simulink model "MotorControl_test"  (R2017a)
settings: Solver=FixedStepDiscrete  StartTime=0.0  StopTime=10.0  RelTol=1e-3
values from neighbouring files (symbols this model uses):
  Enum_MotorState : value not decoded    [MotorControl.sldd]
  PWMValue = 1000.0    [MotorControl.sldd]
undefined symbols (not defined in the file or in its folder): sigbuilder_block
libraries: simulink x5
settings Model: DataDictionary=MotorControl.sldd  Creator=Administrator  LastModifiedBy=Administrator
settings OptimizationCC: DefaultParameterBehavior=Inlined  PassReuseOutputArgsAs=Individual arguments
settings DebuggingCC: ParameterTunabilityLossMsg=error
settings SFSimCC: MATLABDynamicMemAlloc=off
settings RTWCC: SystemTargetFile=ert.tlc  GenCodeOnly=on  TemplateMakefile=ert_default_tmf  Description=Embedded Coder  GenerateReport=on  IncludeHyperlinkInReport=on  LaunchReport=on  GenerateTraceInfo=on  GenerateTraceReport=on  GenerateTraceReportSl=on  GenerateTraceReportSf=on  GenerateTraceReportEml=on
settings CodeAppCC: ForceParamTrailComments=on  IgnoreCustomStorageClasses=off  OperatorAnnotations=on  SimulinkDataObjDesc=on  SFDataObjDesc=on  MATLABFcnDesc=on  InsertBlockDesc=on  MATLABSourceComments=on
settings ERTTargetCC: TargetLangStandard=C99 (ISO)  InlinedParameterPlacement=NonHierarchical  ERTCustomFileTemplate=example_file_process.tlc

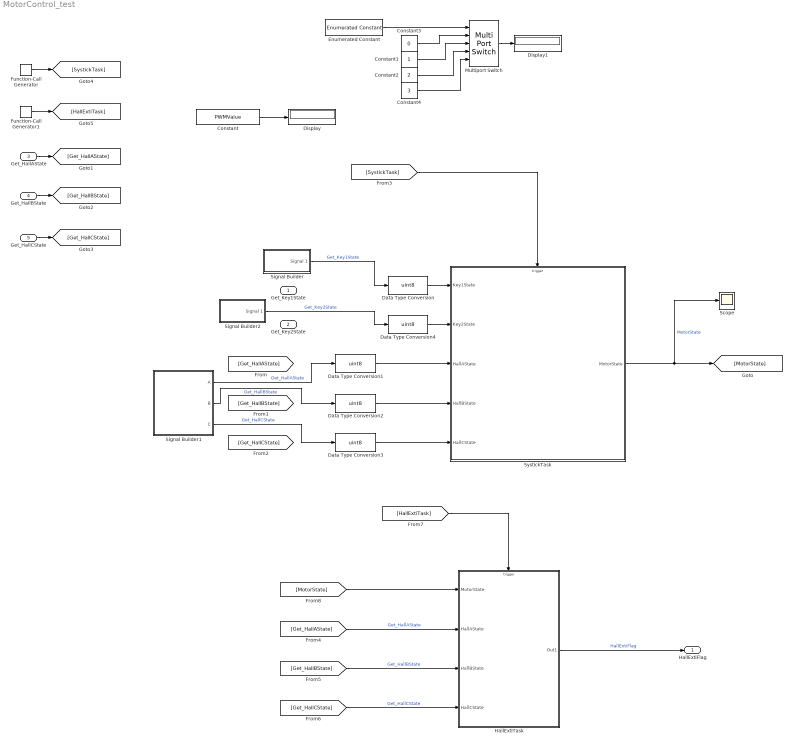
== system MotorControl_test ==
  Get_Key1State : Inport
  Get_Key2State : Inport  Port=2
  Get_HallAState : Inport  Port=3
  Get_HallBState : Inport  Port=4
  Get_HallCState : Inport  Port=5
  Constant : Constant  Value=PWMValue
  Constant1 : Constant  OutDataTypeStr=uint8
  Constant2 : Constant  Value=2  OutDataTypeStr=uint8
  Constant3 : Constant  Value=0  OutDataTypeStr=uint8
  Constant4 : Constant  Value=3  OutDataTypeStr=uint8
  Data Type Conversion{,1..4} (5 alike) : DataTypeConversion  OutDataTypeStr=uint8
  Display : Display
  Display1 : Display
  Enumerated Constant : simulink/Sources/Enumerated Constant  OutDataTypeStr=Enum: Enum_MotorState  Value=Enum_MotorState.Run  SampleTime=inf
      settings: SourceProductName=Simulink
  Function-Call Generator : simulink/Ports & Subsystems/Function-Call Generator  sample_time=0.001  numberOfIterations=1
  Function-Call Generator1 : simulink/Ports & Subsystems/Function-Call Generator  sample_time=1  numberOfIterations=1
  HallExtiTask : Subsystem  TreatAsAtomicUnit=on  RTWFcnName=HallExtiTask
      settings: RTWSystemCode=Nonreusable function  RTWFcnNameOpts=User specified  RTWFileNameOpts=Use function name
  Multiport Switch : MultiPortSwitch  DataPortOrder=Specify indices  DataPortIndices={Enum_MotorState.Init,Enum_MotorState.Stop,Enum_MotorState.Start,Enum_MotorState.Run}
  Scope : Scope
  Signal Builder : Subsystem  Tag=STV Subsys  LoadFcn=sigbuilder_block('load');  StartFcn=sigbuilder_block('start');  StopFcn=sigbuilder_block('stop');  ClipboardFcn=sigbuilder_block('clipboard');  mask(Sigbuilder block){tuvar=[0:10]}
      mask help: Simulink:masks:SigbuilderBlock_MD
      mask init:
      | if ~strcmp(get_param(bdroot(gcbh),'SimulationStatus'),'stopped') tuvar = sigbuilder_block('maskInit'); end
      settings: CopyFcn=sigbuilder_block('copy');  DeleteFcn=sigbuilder_block('delete');  ModelCloseFcn=sigbuilder_block('modelClose');  PreSaveFcn=sigbuilder_block('preSave');  PauseFcn=sigbuilder_block('pause');  ContinueFcn=sigbuilder_block('continue');  NameChangeFcn=sigbuilder_block('namechange');  OpenFcn=sigbuilder_block('open',[437.6 199.2 550.4 400 ]);  CloseFcn=sigbuilder_block('close');
      mask Display: plot(0, 0, 100, 100,[2, 2, 32, 32, 2], [68, 8, 8, 68, 68],[32, 2], [38, 38], [32, 19, 2],[53, 60, 44], [32, 17, 17, 2],[16, 16, 31, 31]);txt = getActiveGroup(gcbh);text(2, 100, txt,'verticalAlignment', 'top');
  Signal Builder1 : Subsystem  Tag=STV Subsys  LoadFcn=sigbuilder_block('load');  StartFcn=sigbuilder_block('start');  StopFcn=sigbuilder_block('stop');  ClipboardFcn=sigbuilder_block('clipboard');  mask(Sigbuilder block){tuvar=[0:10]}
      mask help: Simulink:masks:SigbuilderBlock_MD
      mask init:
      | if ~strcmp(get_param(bdroot(gcbh),'SimulationStatus'),'stopped') tuvar = sigbuilder_block('maskInit'); end
      settings: CopyFcn=sigbuilder_block('copy');  DeleteFcn=sigbuilder_block('delete');  ModelCloseFcn=sigbuilder_block('modelClose');  PreSaveFcn=sigbuilder_block('preSave');  PauseFcn=sigbuilder_block('pause');  ContinueFcn=sigbuilder_block('continue');  NameChangeFcn=sigbuilder_block('namechange');  OpenFcn=sigbuilder_block('open',[437.6 199.2 550.4 400 ]);  CloseFcn=sigbuilder_block('close');
      mask Display: plot(0, 0, 100, 100,[2, 2, 32, 32, 2], [68, 8, 8, 68, 68],[32, 2], [38, 38], [32, 19, 2],[53, 60, 44], [32, 17, 17, 2],[16, 16, 31, 31]);txt = getActiveGroup(gcbh);text(2, 100, txt,'verticalAlignment', 'top');
  Signal Builder2 : Subsystem  Tag=STV Subsys  LoadFcn=sigbuilder_block('load');  StartFcn=sigbuilder_block('start');  StopFcn=sigbuilder_block('stop');  ClipboardFcn=sigbuilder_block('clipboard');  mask(Sigbuilder block){tuvar=[0:10]}
      mask help: Simulink:masks:SigbuilderBlock_MD
      mask init:
      | if ~strcmp(get_param(bdroot(gcbh),'SimulationStatus'),'stopped') tuvar = sigbuilder_block('maskInit'); end
      settings: CopyFcn=sigbuilder_block('copy');  DeleteFcn=sigbuilder_block('delete');  ModelCloseFcn=sigbuilder_block('modelClose');  PreSaveFcn=sigbuilder_block('preSave');  PauseFcn=sigbuilder_block('pause');  ContinueFcn=sigbuilder_block('continue');  NameChangeFcn=sigbuilder_block('namechange');  OpenFcn=sigbuilder_block('open',[437.6 199.2 550.4 400 ]);  CloseFcn=sigbuilder_block('close');
      mask Display: plot(0, 0, 100, 100,[2, 2, 32, 32, 2], [68, 8, 8, 68, 68],[32, 2], [38, 38], [32, 19, 2],[53, 60, 44], [32, 17, 17, 2],[16, 16, 31, 31]);txt = getActiveGroup(gcbh);text(2, 100, txt,'verticalAlignment', 'top');
  SystickTask : Subsystem  TreatAsAtomicUnit=on  RTWFcnName=SystickTask
      settings: RTWSystemCode=Nonreusable function  RTWFcnNameOpts=User specified  RTWFileNameOpts=Use function name
  HallExtiFlag : Outport
  wires:
  SystickTask/1(MotorState) -> Scope/1, [MotorState]  "MotorState"
  HallExtiTask/1(Out1) -> HallExtiFlag/1  "HallExtiFlag"
  [SystickTask] -> SystickTask/Trigger
  Signal Builder1/1(A) -> Data Type Conversion1/1  "Get_HallAState"
  Signal Builder1/3(C) -> Data Type Conversion3/1  "Get_HallCState"
  Signal Builder1/2(B) -> Data Type Conversion2/1  "Get_HallBState"
  Signal Builder2/1(Signal 1) -> Data Type Conversion4/1  "Get_Key2State"
  Signal Builder/1(Signal 1) -> Data Type Conversion/1  "Get_Key1State"
  [HallExtiTask] -> HallExtiTask/Trigger
  [Get_HallCState] -> HallExtiTask/4(HallCState)  "Get_HallCState"
  [Get_HallBState] -> HallExtiTask/3(HallBState)  "Get_HallBState"
  [Get_HallAState] -> HallExtiTask/2(HallAState)  "Get_HallAState"
  [MotorState] -> HallExtiTask/1(MotorState)
  Get_HallAState/1 -> [Get_HallAState]
  Get_HallBState/1 -> [Get_HallBState]
  Get_HallCState/1 -> [Get_HallCState]
  Function-Call Generator/1 -> [SystickTask]
  Function-Call Generator1/1 -> [HallExtiTask]
  Data Type Conversion/1 -> SystickTask/1(Key1State)
  Data Type Conversion1/1 -> SystickTask/3(HallAState)
  Data Type Conversion2/1 -> SystickTask/4(HallBState)
  Data Type Conversion3/1 -> SystickTask/5(HallCState)
  Data Type Conversion4/1 -> SystickTask/2(Key2State)
  Constant/1 -> Display/1
  Constant3/1 -> Multiport Switch/2
  Enumerated Constant/1 -> Multiport Switch/1
  Constant1/1 -> Multiport Switch/3
  Constant2/1 -> Multiport Switch/4
  Constant4/1 -> Multiport Switch/5
  Multiport Switch/1 -> Display1/1

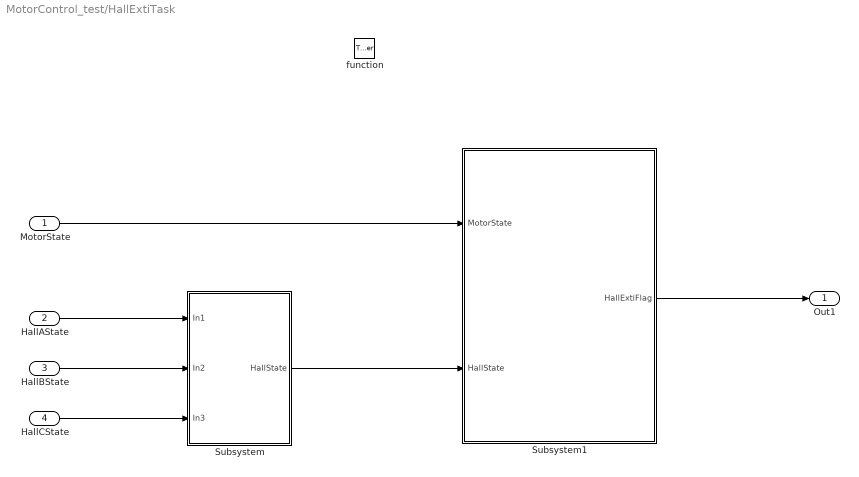
== system MotorControl_test/HallExtiTask ==
  MotorState : Inport
  HallAState : Inport  Port=2
  HallBState : Inport  Port=3
  HallCState : Inport  Port=4
  function : TriggerPort  TriggerType=function-call  VariantControl=Variant
  Subsystem : Subsystem
  Subsystem1 : Subsystem
  Out1 : Outport
  wires:
  HallBState/1 -> Subsystem/2(In2)
  HallAState/1 -> Subsystem/1(In1)
  HallCState/1 -> Subsystem/3(In3)
  MotorState/1 -> Subsystem1/1(MotorState)
  Subsystem/1(HallState) -> Subsystem1/2(HallState)
  Subsystem1/1(HallExtiFlag) -> Out1/1

== system MotorControl_test/Signal Builder ==
  Demux : Demux  Tag=STV Demux  Outputs=1
  FromWs : FromWorkspace  Tag=STV FromWs  VariableName=tuvar  SampleTime=0
      SigBuilderData=|
      | common.afterFinalStr = 'Extrapolate'
      | common.sampleTime = 0
      | dataSet.timeRange = [0 10]
      | dataSet.name = 'Group 1'
      | sbobj.Groups.Name = 'Group 1'
      | sbobj.Groups.Signals.Name = 'Signal 1'
      | sbobj.Groups.Signals.XData = [0 4 4 6 6 10]
      | sbobj.Groups.Signals.YData = [0 0 1 1 0 0]
  Signal 1 : Outport  Tag=STV Outport
  wires:
  Demux/1 -> Signal 1/1
  FromWs/1 -> Demux/1

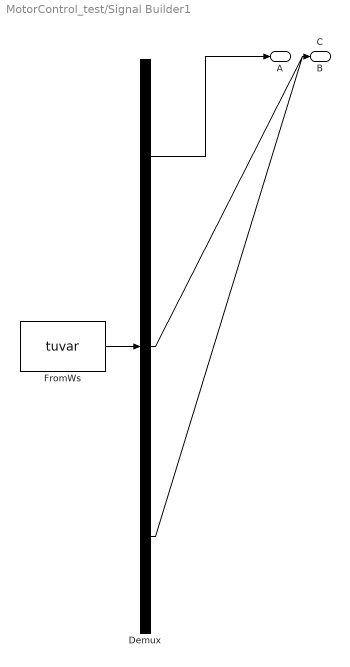
== system MotorControl_test/Signal Builder1 ==
  Demux : Demux  Tag=STV Demux  Outputs=3
  FromWs : FromWorkspace  Tag=STV FromWs  VariableName=tuvar  SampleTime=0
      SigBuilderData=|
      | common.afterFinalStr = 'Extrapolate'
      | common.sampleTime = 0
      | dataSet.timeRange = [0 7.999]
      | dataSet.name = 'Sheet1'
      | sbobj.Groups.Name = 'Sheet1'
      | sbobj.Groups.Signals(1).Name = 'A'
      | sbobj.Groups.Signals(1).XData = [0 4.999 5 5.499 5.5 5.999 6 6.499 6.5 6.999 7 7.499 7.5 7.999]
      | sbobj.Groups.Signals(1).YData = [0 0 1 1 1 1 1 1 0 0 0 0 0 0]
      | sbobj.Groups.Signals(2).Name = 'B'
      | sbobj.Groups.Signals(2).XData = [0 4.999 5 5.499 5.5 5.999 6 6.499 6.5 6.999 7 7.499 7.5 7.999]
      | sbobj.Groups.Signals(2).YData = [0 0 0 0 0 0 1 1 1 1 1 1 0 0]
      | sbobj.Groups.Signals(3).Name = 'C'
      | sbobj.Groups.Signals(3).XData = [0 4.999 5 5.499 5.5 5.999 6 6.499 6.5 6.999 7 7.499 7.5 7.999]
      | sbobj.Groups.Signals(3).YData = [0 0 1 1 0 0 0 0 0 0 1 1 1 1]
      | sbobj.Groups.TimeRange = [0 7.999]
  A : Outport  Tag=STV Outport
  B : Outport  Tag=STV Outport  Port=2
  C : Outport  Tag=STV Outport  Port=3
  wires:
  FromWs/1 -> Demux/1
  Demux/1 -> A/1
  Demux/2 -> B/1
  Demux/3 -> C/1

== system MotorControl_test/Signal Builder2 ==
  Demux : Demux  Tag=STV Demux  Outputs=1
  FromWs : FromWorkspace  Tag=STV FromWs  VariableName=tuvar  SampleTime=0
      SigBuilderData=|
      | common.afterFinalStr = 'Extrapolate'
      | common.sampleTime = 0
      | dataSet.timeRange = [0 10]
      | dataSet.name = 'Group 1'
      | sbobj.Groups.Name = 'Group 1'
      | sbobj.Groups.Signals.Name = 'Signal 1'
      | sbobj.Groups.Signals.XData = [0 9 9 9.76 9.76 10]
      | sbobj.Groups.Signals.YData = [0 0 1 1 0 0]
  Signal 1 : Outport  Tag=STV Outport
  wires:
  FromWs/1 -> Demux/1
  Demux/1 -> Signal 1/1

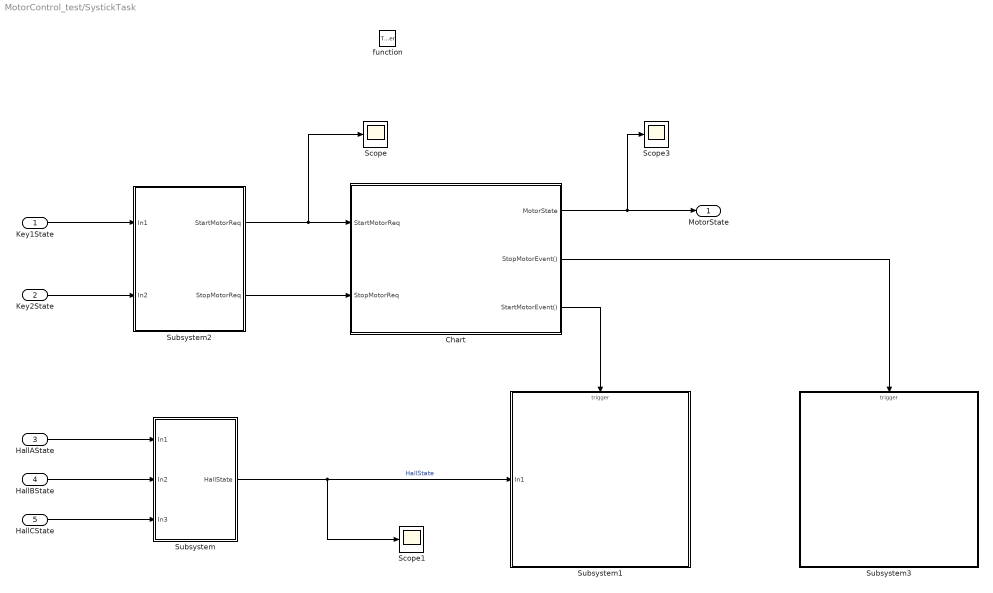
== system MotorControl_test/SystickTask ==
  Key1State : Inport
  Key2State : Inport  Port=2
  HallAState : Inport  Port=3
  HallBState : Inport  Port=4
  HallCState : Inport  Port=5
  function : TriggerPort  TriggerType=function-call  VariantControl=Variant
  Chart : Stateflow chart  TreatAsAtomicUnit=on
  Scope : Scope
  Scope1 : Scope
  Scope3 : Scope
  Subsystem : Subsystem
  Subsystem1 : Subsystem
  Subsystem2 : Subsystem
  Subsystem3 : Subsystem
      settings: RTWSystemCode=Nonreusable function
  MotorState : Outport
  wires:
  Key1State/1 -> Subsystem2/1(In1)
  Key2State/1 -> Subsystem2/2(In2)
  Subsystem2/1(StartMotorReq) -> Scope/1, Chart/1(StartMotorReq)
  Subsystem2/2(StopMotorReq) -> Chart/2(StopMotorReq)
  Chart/1(MotorState) -> Scope3/1, MotorState/1
  HallAState/1 -> Subsystem/1(In1)
  HallBState/1 -> Subsystem/2(In2)
  HallCState/1 -> Subsystem/3(In3)
  Subsystem/1(HallState) -> Subsystem1/1(In1), Scope1/1  "HallState"
  Chart/2(StopMotorEvent()) -> Subsystem3/Trigger
  Chart/3(StartMotorEvent()) -> Subsystem1/Trigger

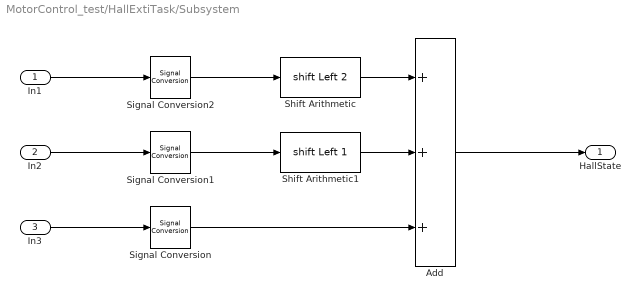
== system MotorControl_test/HallExtiTask/Subsystem ==
  In1 : Inport
  In2 : Inport  Port=2
  In3 : Inport  Port=3
  Add : Sum  Inputs=+++
  Shift Arithmetic : ArithShift  BitShiftNumber=2  BitShiftDirection=Left
  Shift Arithmetic1 : ArithShift  BitShiftNumber=1  BitShiftDirection=Left
  Signal Conversion : SignalConversion  OverrideOpt=off
  Signal Conversion1 : SignalConversion  OverrideOpt=off
  Signal Conversion2 : SignalConversion  OverrideOpt=on
  HallState : Outport
  wires:
  Add/1 -> HallState/1
  Signal Conversion/1 -> Add/3
  In3/1 -> Signal Conversion/1
  Signal Conversion1/1 -> Shift Arithmetic1/1
  Signal Conversion2/1 -> Shift Arithmetic/1
  Shift Arithmetic/1 -> Add/1
  In1/1 -> Signal Conversion2/1
  In2/1 -> Signal Conversion1/1
  Shift Arithmetic1/1 -> Add/2

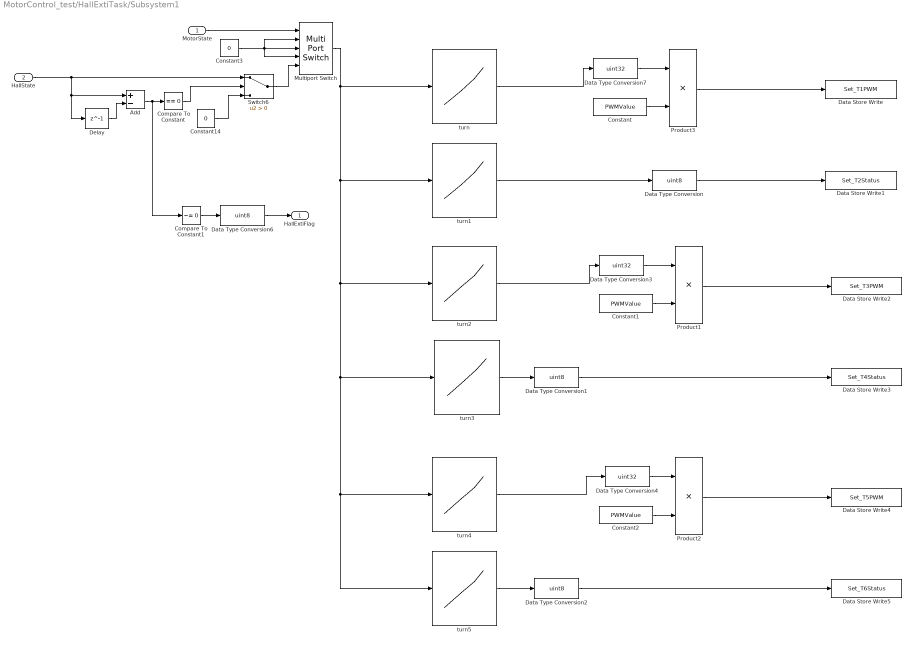
== system MotorControl_test/HallExtiTask/Subsystem1 ==
  MotorState : Inport
  HallState : Inport  Port=2
  Add : Sum  Inputs=+-
  Compare To Constant : simulink/Logic and Bit Operations/Compare To Constant  relop===  const=0  OutDataTypeStr=boolean
  Compare To Constant1 : simulink/Logic and Bit Operations/Compare To Constant  relop=~=  const=0  OutDataTypeStr=boolean
  Constant : Constant  Value=PWMValue
  Constant1 : Constant  Value=PWMValue
  Constant14 : Constant  Value=0  OutDataTypeStr=uint8
  Constant2 : Constant  Value=PWMValue
  Constant3 : Constant  Value=0  OutDataTypeStr=uint8
  Data Store Write : DataStoreWrite  DataStoreName=Set_T1PWM
  Data Store Write1 : DataStoreWrite  DataStoreName=Set_T2Status
  Data Store Write2 : DataStoreWrite  DataStoreName=Set_T3PWM
  Data Store Write3 : DataStoreWrite  DataStoreName=Set_T4Status
  Data Store Write4 : DataStoreWrite  DataStoreName=Set_T5PWM
  Data Store Write5 : DataStoreWrite  DataStoreName=Set_T6Status
  Data Type Conversion{,1..2,6} (4 alike) : DataTypeConversion  OutDataTypeStr=uint8
  Data Type Conversion3 : DataTypeConversion  OutDataTypeStr=uint32
  Data Type Conversion4 : DataTypeConversion  OutDataTypeStr=uint32
  Data Type Conversion7 : DataTypeConversion  OutDataTypeStr=uint32
  Delay : Delay  DelayLength=1  InitialCondition=0
  Multiport Switch : MultiPortSwitch  DataPortOrder=Specify indices  DataPortIndices={Enum_MotorState.Init,Enum_MotorState.Stop,Enum_MotorState.Start,Enum_MotorState.Run}
  Product1 : Product  OutDataTypeStr=uint32
  Product2 : Product  OutDataTypeStr=uint32
  Product3 : Product  OutDataTypeStr=uint32
  Switch6 : Switch  Criteria=u2 > Threshold
  turn : Lookup_n-D  NumberOfTableDimensions=1  BreakpointsForDimension1=[0 1 2 3 4 5 6]  Table=[0 0 0 0 1 1 0]  InterpMethod=Nearest  InternalRulePriority=Speed  RndMeth=Simplest  InputSameDT=on
  turn1 : Lookup_n-D  NumberOfTableDimensions=1  BreakpointsForDimension1=[0 1 2 3 4 5 6]  Table=[0 0 1 1 0 0 0 ]  InterpMethod=Nearest  InternalRulePriority=Speed  RndMeth=Simplest  InputSameDT=on
  turn2 : Lookup_n-D  NumberOfTableDimensions=1  BreakpointsForDimension1=[0 1 2 3 4 5 6]  Table=[0 0 1 0 0 0 1]  InterpMethod=Nearest  InternalRulePriority=Speed  RndMeth=Simplest  InputSameDT=on
  turn3 : Lookup_n-D  NumberOfTableDimensions=1  BreakpointsForDimension1=[0 1 2 3 4 5 6]  Table=[0 1 0 0 0 1 0]  InterpMethod=Nearest  InternalRulePriority=Speed  RndMeth=Simplest  InputSameDT=on
  turn4 : Lookup_n-D  NumberOfTableDimensions=1  BreakpointsForDimension1=[0 1 2 3 4 5 6]  Table=[0 1 0 1 0 0 0]  InterpMethod=Nearest  InternalRulePriority=Speed  RndMeth=Simplest  InputSameDT=on
  turn5 : Lookup_n-D  NumberOfTableDimensions=1  BreakpointsForDimension1=[0 1 2 3 4 5 6]  Table=[0 0 0 0 1 0 1]  InterpMethod=Nearest  InternalRulePriority=Speed  RndMeth=Simplest  InputSameDT=on
  HallExtiFlag : Outport
  wires:
  Constant2/1 -> Product2/2
  turn5/1 -> Data Type Conversion2/1
  Product2/1 -> Data Store Write4/1
  Data Type Conversion2/1 -> Data Store Write5/1
  turn4/1 -> Data Type Conversion4/1
  turn1/1 -> Data Type Conversion/1
  Multiport Switch/1 -> turn/1, turn4/1, turn5/1, turn3/1, turn2/1, turn1/1
  Data Type Conversion/1 -> Data Store Write1/1
  turn3/1 -> Data Type Conversion1/1
  Constant1/1 -> Product1/2
  turn2/1 -> Data Type Conversion3/1
  Product1/1 -> Data Store Write2/1
  Data Type Conversion1/1 -> Data Store Write3/1
  Product3/1 -> Data Store Write/1
  turn/1 -> Data Type Conversion7/1
  Constant/1 -> Product3/2
  Compare To Constant/1 -> Switch6/2
  Delay/1 -> Add/2
  HallState/1 -> Add/1, Delay/1, Switch6/1
  Constant14/1 -> Switch6/3
  Add/1 -> Compare To Constant1/1, Compare To Constant/1
  MotorState/1 -> Multiport Switch/1
  Switch6/1 -> Multiport Switch/5
  Constant3/1 -> Multiport Switch/2, Multiport Switch/3, Multiport Switch/4
  Compare To Constant1/1 -> Data Type Conversion6/1
  Data Type Conversion6/1 -> HallExtiFlag/1
  Data Type Conversion7/1 -> Product3/1
  Data Type Conversion3/1 -> Product1/1
  Data Type Conversion4/1 -> Product2/1

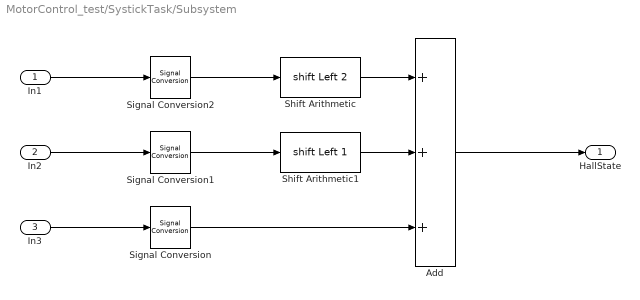
== system MotorControl_test/SystickTask/Subsystem ==
  In1 : Inport
  In2 : Inport  Port=2
  In3 : Inport  Port=3
  Add : Sum  Inputs=+++
  Shift Arithmetic : ArithShift  BitShiftNumber=2  BitShiftDirection=Left
  Shift Arithmetic1 : ArithShift  BitShiftNumber=1  BitShiftDirection=Left
  Signal Conversion : SignalConversion  OverrideOpt=off
  Signal Conversion1 : SignalConversion  OverrideOpt=off
  Signal Conversion2 : SignalConversion  OverrideOpt=off
  HallState : Outport
  wires:
  Add/1 -> HallState/1
  Signal Conversion/1 -> Add/3
  In3/1 -> Signal Conversion/1
  Signal Conversion1/1 -> Shift Arithmetic1/1
  Signal Conversion2/1 -> Shift Arithmetic/1
  Shift Arithmetic/1 -> Add/1
  In1/1 -> Signal Conversion2/1
  In2/1 -> Signal Conversion1/1
  Shift Arithmetic1/1 -> Add/2

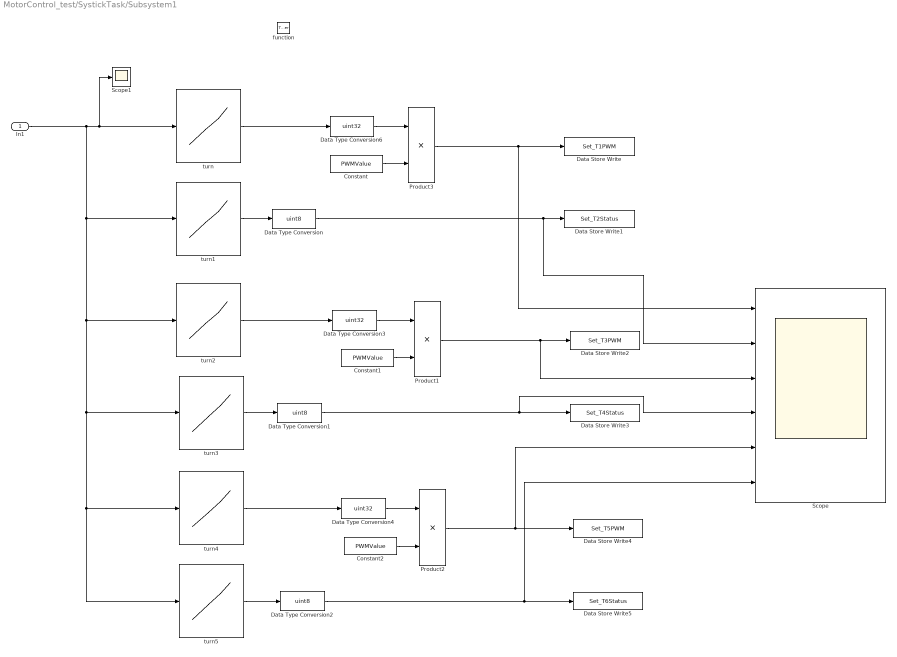
== system MotorControl_test/SystickTask/Subsystem1 ==
  In1 : Inport
  function : TriggerPort  TriggerType=function-call  VariantControl=Variant
  Constant : Constant  Value=PWMValue
  Constant1 : Constant  Value=PWMValue
  Constant2 : Constant  Value=PWMValue
  Data Store Write : DataStoreWrite  DataStoreName=Set_T1PWM
  Data Store Write1 : DataStoreWrite  DataStoreName=Set_T2Status
  Data Store Write2 : DataStoreWrite  DataStoreName=Set_T3PWM
  Data Store Write3 : DataStoreWrite  DataStoreName=Set_T4Status
  Data Store Write4 : DataStoreWrite  DataStoreName=Set_T5PWM
  Data Store Write5 : DataStoreWrite  DataStoreName=Set_T6Status
  Data Type Conversion : DataTypeConversion  OutDataTypeStr=uint8
  Data Type Conversion1 : DataTypeConversion  OutDataTypeStr=uint8
  Data Type Conversion2 : DataTypeConversion  OutDataTypeStr=uint8
  Data Type Conversion3 : DataTypeConversion  OutDataTypeStr=uint32
  Data Type Conversion4 : DataTypeConversion  OutDataTypeStr=uint32
  Data Type Conversion6 : DataTypeConversion  OutDataTypeStr=uint32
  Product1 : Product  OutDataTypeStr=uint32
  Product2 : Product  OutDataTypeStr=uint32
  Product3 : Product  OutDataTypeStr=uint32
  Scope : Scope  NumInputPorts=6
  Scope1 : Scope
  turn : Lookup_n-D  NumberOfTableDimensions=1  BreakpointsForDimension1=[1 2 3 4 5 6]  Table=[0 0 0 1 1 0]  InterpMethod=Nearest  InternalRulePriority=Speed  RndMeth=Simplest  InputSameDT=on
  turn1 : Lookup_n-D  NumberOfTableDimensions=1  BreakpointsForDimension1=[1 2 3 4 5 6]  Table=[0 1 1 0 0 0 ]  InterpMethod=Nearest  InternalRulePriority=Speed  RndMeth=Simplest  InputSameDT=on
  turn2 : Lookup_n-D  NumberOfTableDimensions=1  BreakpointsForDimension1=[1 2 3 4 5 6]  Table=[0 1 0 0 0 1]  InterpMethod=Nearest  InternalRulePriority=Speed  RndMeth=Simplest  InputSameDT=on
  turn3 : Lookup_n-D  NumberOfTableDimensions=1  BreakpointsForDimension1=[1 2 3 4 5 6]  Table=[1 0 0 0 1 0]  InterpMethod=Nearest  InternalRulePriority=Speed  RndMeth=Simplest  InputSameDT=on
  turn4 : Lookup_n-D  NumberOfTableDimensions=1  BreakpointsForDimension1=[1 2 3 4 5 6]  Table=[1 0 1 0 0 0]  InterpMethod=Nearest  InternalRulePriority=Speed  RndMeth=Simplest  InputSameDT=on
  turn5 : Lookup_n-D  NumberOfTableDimensions=1  BreakpointsForDimension1=[1 2 3 4 5 6]  Table=[0 0 0 1 0 1]  InterpMethod=Nearest  InternalRulePriority=Speed  RndMeth=Simplest  InputSameDT=on
  wires:
  Constant2/1 -> Product2/2
  turn5/1 -> Data Type Conversion2/1
  Product2/1 -> Scope/5, Data Store Write4/1
  Data Type Conversion2/1 -> Scope/6, Data Store Write5/1
  turn4/1 -> Data Type Conversion4/1
  turn1/1 -> Data Type Conversion/1
  In1/1 -> turn1/1, turn3/1, turn4/1, turn5/1, turn2/1, Scope1/1, turn/1
  Data Type Conversion/1 -> Scope/2, Data Store Write1/1
  turn3/1 -> Data Type Conversion1/1
  Constant1/1 -> Product1/2
  turn2/1 -> Data Type Conversion3/1
  Product1/1 -> Scope/3, Data Store Write2/1
  Data Type Conversion1/1 -> Scope/4, Data Store Write3/1
  Product3/1 -> Scope/1, Data Store Write/1
  turn/1 -> Data Type Conversion6/1
  Constant/1 -> Product3/2
  Data Type Conversion6/1 -> Product3/1
  Data Type Conversion3/1 -> Product1/1
  Data Type Conversion4/1 -> Product2/1

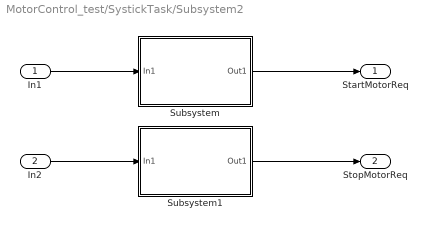
== system MotorControl_test/SystickTask/Subsystem2 ==
  In1 : Inport
  In2 : Inport  Port=2
  Subsystem : Subsystem
  Subsystem1 : Subsystem
  StartMotorReq : Outport
  StopMotorReq : Outport  Port=2
  wires:
  Subsystem/1(Out1) -> StartMotorReq/1
  Subsystem1/1(Out1) -> StopMotorReq/1
  In2/1 -> Subsystem1/1(In1)
  In1/1 -> Subsystem/1(In1)

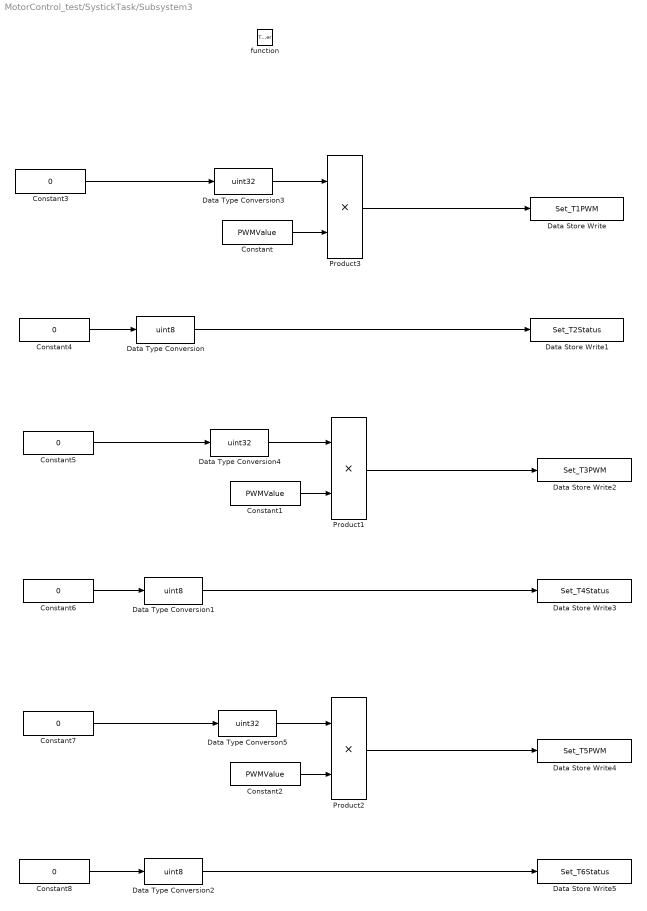
== system MotorControl_test/SystickTask/Subsystem3 ==
  function : TriggerPort  TriggerType=function-call  VariantControl=Variant
  Constant : Constant  Value=PWMValue
  Constant1 : Constant  Value=PWMValue
  Constant2 : Constant  Value=PWMValue
  Constant{3..8} (6 alike) : Constant  Value=0
  Data Store Write : DataStoreWrite  DataStoreName=Set_T1PWM
  Data Store Write1 : DataStoreWrite  DataStoreName=Set_T2Status
  Data Store Write2 : DataStoreWrite  DataStoreName=Set_T3PWM
  Data Store Write3 : DataStoreWrite  DataStoreName=Set_T4Status
  Data Store Write4 : DataStoreWrite  DataStoreName=Set_T5PWM
  Data Store Write5 : DataStoreWrite  DataStoreName=Set_T6Status
  Data Type Conversion : DataTypeConversion  OutDataTypeStr=uint8
  Data Type Conversion1 : DataTypeConversion  OutDataTypeStr=uint8
  Data Type Conversion2 : DataTypeConversion  OutDataTypeStr=uint8
  Data Type Conversion3 : DataTypeConversion  OutDataTypeStr=uint32
  Data Type Conversion4 : DataTypeConversion  OutDataTypeStr=uint32
  Data Type Converson5 : DataTypeConversion  OutDataTypeStr=uint32
  Product1 : Product  OutDataTypeStr=uint32
  Product2 : Product  OutDataTypeStr=uint32
  Product3 : Product  OutDataTypeStr=uint32
  wires:
  Constant/1 -> Product3/2
  Constant3/1 -> Data Type Conversion3/1
  Product3/1 -> Data Store Write/1
  Data Type Conversion1/1 -> Data Store Write3/1
  Product1/1 -> Data Store Write2/1
  Constant5/1 -> Data Type Conversion4/1
  Constant1/1 -> Product1/2
  Constant6/1 -> Data Type Conversion1/1
  Data Type Conversion/1 -> Data Store Write1/1
  Constant4/1 -> Data Type Conversion/1
  Constant7/1 -> Data Type Converson5/1
  Data Type Conversion2/1 -> Data Store Write5/1
  Product2/1 -> Data Store Write4/1
  Constant8/1 -> Data Type Conversion2/1
  Constant2/1 -> Product2/2
  Data Type Conversion3/1 -> Product3/1
  Data Type Conversion4/1 -> Product1/1
  Data Type Converson5/1 -> Product2/1

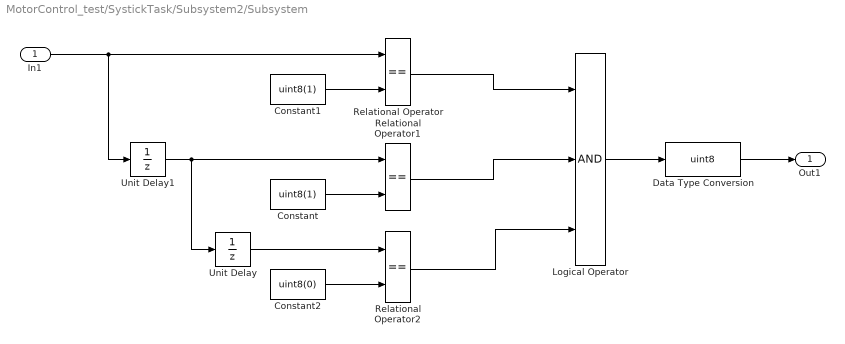
== system MotorControl_test/SystickTask/Subsystem2/Subsystem ==
  In1 : Inport
  Constant : Constant  Value=uint8(1)
  Constant1 : Constant  Value=uint8(1)
  Constant2 : Constant  Value=uint8(0)
  Data Type Conversion : DataTypeConversion  OutDataTypeStr=uint8
  Logical Operator : Logic  Inputs=3  AllPortsSameDT=off  OutDataTypeStr=boolean
  Relational Operator : RelationalOperator  Operator===  OutDataTypeStr=boolean  RndMeth=Simplest
  Relational Operator1 : RelationalOperator  Operator===  OutDataTypeStr=boolean  RndMeth=Simplest
  Relational Operator2 : RelationalOperator  Operator===  OutDataTypeStr=boolean  RndMeth=Simplest
  Unit Delay : UnitDelay  SampleTime=-1
  Unit Delay1 : UnitDelay  SampleTime=-1
  Out1 : Outport
  wires:
  Constant2/1 -> Relational Operator2/2
  Unit Delay1/1 -> Unit Delay/1, Relational Operator1/1
  Constant1/1 -> Relational Operator/2
  Relational Operator2/1 -> Logical Operator/3
  Relational Operator1/1 -> Logical Operator/2
  Relational Operator/1 -> Logical Operator/1
  Constant/1 -> Relational Operator1/2
  In1/1 -> Unit Delay1/1, Relational Operator/1
  Unit Delay/1 -> Relational Operator2/1
  Logical Operator/1 -> Data Type Conversion/1
  Data Type Conversion/1 -> Out1/1

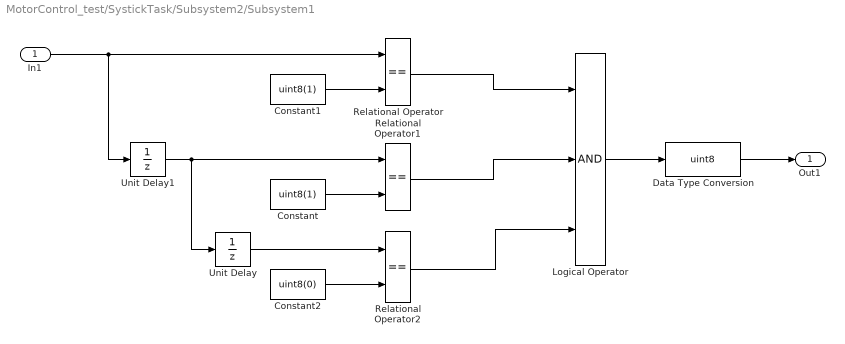
== system MotorControl_test/SystickTask/Subsystem2/Subsystem1 ==
  In1 : Inport
  Constant : Constant  Value=uint8(1)
  Constant1 : Constant  Value=uint8(1)
  Constant2 : Constant  Value=uint8(0)
  Data Type Conversion : DataTypeConversion  OutDataTypeStr=uint8
  Logical Operator : Logic  Inputs=3  AllPortsSameDT=off  OutDataTypeStr=boolean
  Relational Operator : RelationalOperator  Operator===  OutDataTypeStr=boolean  RndMeth=Simplest
  Relational Operator1 : RelationalOperator  Operator===  OutDataTypeStr=boolean  RndMeth=Simplest
  Relational Operator2 : RelationalOperator  Operator===  OutDataTypeStr=boolean  RndMeth=Simplest
  Unit Delay : UnitDelay  SampleTime=-1
  Unit Delay1 : UnitDelay  SampleTime=-1
  Out1 : Outport
  wires:
  Data Type Conversion/1 -> Out1/1
  Logical Operator/1 -> Data Type Conversion/1
  Unit Delay/1 -> Relational Operator2/1
  In1/1 -> Relational Operator/1, Unit Delay1/1
  Constant/1 -> Relational Operator1/2
  Relational Operator/1 -> Logical Operator/1
  Relational Operator1/1 -> Logical Operator/2
  Relational Operator2/1 -> Logical Operator/3
  Constant1/1 -> Relational Operator/2
  Unit Delay1/1 -> Relational Operator1/1, Unit Delay/1
  Constant2/1 -> Relational Operator2/2

== stateflow chart MotorControl_test/SystickTask/Chart ==
  state Init
    en:
    MotorState = Enum_MotorState.Init;
  state Start
    en:
    MotorState = Enum_MotorState.Start;
    StartCount = 0;
    StartMotorEvent;
    du:
    StartCount = StartCount + 1;
  state Stop
    en:
    MotorState = Enum_MotorState.Stop;
    StopMotorEvent;
  state Run
    en:
    MotorState = Enum_MotorState.Run;
    StartCount = 0;
  (default) -> Init
  Init -> Start : [StartMotorReq == 1]
  Stop -> Start : [StartMotorReq == 1]
  Start -> Stop [order 2] : [StopMotorReq == 1]
  Start -> Run [order 1] : [StartCount == 10]
  Run -> Stop : [StopMotorReq == 1]
  data: StartMotorReq input; StopMotorReq input; MotorState output; StartCount local
  events: StopMotorEvent output FUNCTION_CALL_EVENT; StartMotorEvent output FUNCTION_CALL_EVENT
